simulink subsystem "Final_Project"  (R2024a)
settings: Solver=VariableStepAuto  StartTime=0.0  StopTime=10.0  RelTol=1e-3
undefined symbols (not defined in the file or in its folder): waypoints
libraries: CarMaker4SL x82
(part 4 of 4)

== matlab function Final_Project/Lib_Driving/Subsystem/MATLAB Function2 ==
  data: lat_err input; steer output; head_err input; curve_abs input; ego_v input; target_speed input; front_dist input; front_v input; mode input; lchg_done input; accel output; front_dist_lock output; park_cmd input; ego input
function [steer, accel, front_dist_lock] = controller(...
    lat_err, head_err, curve_abs, ego_v, target_speed, ...
    front_dist, front_v, mode, lchg_done, park_cmd, ego)
%#codegen

    % ============================================================
    % 기본 상수
    % ============================================================
    TS           = 0.01;
    STEER_LIM    = 0.58;
    MAX_SPEED    = 50.0;
    MODE_LCHG    = int32(1);
    MODE_PARK    = int32(2);
    KAPPA_EPS    = 1e-4;
    SPD_DEADBAND = 0.3;

    % ============================================================
    % Ego position
    % ============================================================
    ego_x = ego.Car_Fr1_tx;
    ego_y = ego.Car_Fr1_ty;

    % ============================================================
    % Parking waypoints
    % ============================================================
    L4_X     = -46.856;  L4_Y     = 15.842;
    L5_END_X =  2.617;   L5_END_Y = -35.0;

    dist_l4     = sqrt((ego_x - L4_X)^2     + (ego_y - L4_Y)^2);
    dist_to_end = sqrt((ego_x - L5_END_X)^2 + (ego_y - L5_END_Y)^2);

    % ============================================================
    % 파라미터 정의: 일반 주행 / 주차 진입
    %
    % 일반 주행부는 오류 고친 코드의 공격적인 주행 파라미터를 반영
    % 주차 진입부는 기존 주차장 버전의 저속 안정 파라미터 유지
    % ============================================================
    K_STANLEY_NRM  = 0.88;   K_STANLEY_PRK  = 0.20;
    KP_HEAD_NRM    = 0.90;   KP_HEAD_PRK    = 0.50;
    LOOK_FRONT_NRM = calcLookFront(ego_v);  LOOK_FRONT_PRK = 10.0;
    ALAT_NRM       = 3.50;   ALAT_PRK       = 1.50; %허용 횡가속도
    ATOT_NRM       = 4.00;   ATOT_PRK       = 2.00;
    MCSPD_NRM      = 7.00;   MCSPD_PRK      = 1.00;
    VREF_A_NRM     = 50.0;   VREF_A_PRK     = 2.00;
    VREF_D_NRM     = 100.0;  VREF_D_PRK     = 5.00;
    JERK_U_NRM     = 50.0;   JERK_U_PRK     = 3.00;
    JERK_D_NRM     = 60.0;   JERK_D_PRK     = 5.00;
    AMAX_NRM       = 10.0;   AMAX_PRK       = 3.00;
    DMAX_NRM       = 10.0;   DMAX_PRK       = 5.00;

    % ============================================================
    % park_cmd에 따른 파라미터 보간
    % L4에 가까워질수록 일반 주행 -> 주차 진입 파라미터로 부드럽게 전환
    % ============================================================
    FADE_FAR  = 50.0;
    FADE_NEAR = 20.0;

    if park_cmd == int32(1)
        if dist_l4 >= FADE_FAR
            r = 0.0;
        elseif dist_l4 <= FADE_NEAR
            r = 1.0;
        else
            r = (FADE_FAR - dist_l4) / (FADE_FAR - FADE_NEAR);
        end
    else
        r = 0.0;
    end

    K_STANLEY       = K_STANLEY_NRM  + r * (K_STANLEY_PRK  - K_STANLEY_NRM);
    KP_HEAD         = KP_HEAD_NRM    + r * (KP_HEAD_PRK    - KP_HEAD_NRM);
    LOOK_FRONT      = LOOK_FRONT_NRM + r * (LOOK_FRONT_PRK - LOOK_FRONT_NRM);
    A_LAT_LIMIT     = ALAT_NRM       + r * (ALAT_PRK       - ALAT_NRM);
    A_TOTAL_LIMIT   = ATOT_NRM       + r * (ATOT_PRK       - ATOT_NRM);
    MIN_CURVE_SPEED = MCSPD_NRM      + r * (MCSPD_PRK      - MCSPD_NRM);
    V_REF_ACCEL     = VREF_A_NRM     + r * (VREF_A_PRK     - VREF_A_NRM);
    V_REF_DECEL     = VREF_D_NRM     + r * (VREF_D_PRK     - VREF_D_NRM);
    JERK_UP         = JERK_U_NRM     + r * (JERK_U_PRK     - JERK_U_NRM);
    JERK_DOWN       = JERK_D_NRM     + r * (JERK_D_PRK     - JERK_D_NRM);
    ACCEL_MAX_BASE  = AMAX_NRM       + r * (AMAX_PRK       - AMAX_NRM);
    DECEL_MAX_BASE  = DMAX_NRM       + r * (DMAX_PRK       - DMAX_NRM);

    % ============================================================
    % 목표속도 결정
    % ============================================================
    if park_cmd == int32(1)

        DECEL_DIST = 25.0;
        STOP_DIST  =  2.0;

        if mode == MODE_PARK

            if dist_to_end < STOP_DIST
                ts = 0.0;
            elseif dist_to_end < DECEL_DIST
                ts = 1.4 * (dist_to_end / DECEL_DIST);
            else
                ts = 1.4;
            end

        elseif dist_l4 > FADE_NEAR

            spd_far  = 8.3;
            spd_near = 2.8;

            if dist_l4 >= FADE_FAR
                ts = spd_far;
            else
                ts = spd_far + (spd_near - spd_far) * r;
            end

        else

            ts = 2.8;

        end

    else

        ts = target_speed;

        % target_speed가 20보다 크면 km/h라고 보고 m/s로 변환
        if ts > 20.0
            ts = ts / 3.6;
        end

    end

    if ts > MAX_SPEED
        ts = MAX_SPEED;
    end

    if ts < 0.0
        ts = 0.0;
    end

    % ============================================================
    % persistent
    % ============================================================
    persistent desired_v_p accel_p did_init

    if isempty(did_init)
        desired_v_p = ego_v;
        accel_p     = 0.0;
        did_init    = true;
    end

    % ============================================================
    % 1. Stanley 조향
    % ============================================================
    v_safe = ego_v;

    if v_safe < 1.0
        v_safe = 1.0;
    end

    steer = KP_HEAD * head_err - atan2(K_STANLEY * lat_err, v_safe);

    if steer > STEER_LIM
        steer = STEER_LIM;
    elseif steer < -STEER_LIM
        steer = -STEER_LIM;
    end

    % ============================================================
    % 1-1. 끝점 추가 좌회전 블렌드
    % park_cmd=1, MODE_PARK, 끝점 5m 이내에서만 적용
    % ============================================================
    EXTRA_DIST = 5.0;
    EXTRA_RAD  = pi / 3.0;   % 60 deg

    if park_cmd == int32(1) && mode == MODE_PARK
        if dist_to_end < EXTRA_DIST && dist_to_end > 0.0
            blend = 1.0 - (dist_to_end / EXTRA_DIST);
            steer = steer + blend * EXTRA_RAD;

            % 끝점 구간만 추가 조향 허용
            if steer > EXTRA_RAD
                steer = EXTRA_RAD;
            elseif steer < -EXTRA_RAD
                steer = -EXTRA_RAD;
            end
        end
    end

    % ============================================================
    % 2. 곡률 기반 목표속도 제한
    % ============================================================
    desired_v_raw = ts;

    if curve_abs > KAPPA_EPS

        v_curve = sqrt(A_LAT_LIMIT / curve_abs);

        if v_curve < MIN_CURVE_SPEED
            v_curve = MIN_CURVE_SPEED;
        end

        if v_curve < desired_v_raw
            desired_v_raw = v_curve;
        end
    end

    % ============================================================
    % 3. ACC 앞차 감속
    % 주차 진입 중에는 비활성화
    % ============================================================
    % if park_cmd ~= int32(1)
    if mode ~= MODE_PARK

        if front_dist < LOOK_FRONT

            time_gap = 2.0;
            ACC_GAIN = 0.5;

            safe_v = front_v + (front_dist - time_gap * ego_v) * ACC_GAIN;

            if safe_v < desired_v_raw
                desired_v_raw = safe_v;
            end
        end
    end

    if desired_v_raw < 0.0
        desired_v_raw = 0.0;
    end

    % ============================================================
    % 4. 목표속도 변화율 제한
    % ============================================================
    dv = desired_v_raw - desired_v_p;

    max_dv_up = V_REF_ACCEL * TS;
    max_dv_dn = V_REF_DECEL * TS;

    if dv > max_dv_up
        desired_v_p = desired_v_p + max_dv_up;
    elseif dv < -max_dv_dn
        desired_v_p = desired_v_p - max_dv_dn;
    else
        desired_v_p = desired_v_raw;
    end

    desired_v = desired_v_p;

    % ============================================================
    % 5. 가감속
    % 주차 구간: 비례제어
    % 일반 구간: 기록 단축용 Bang-Bang
    % ============================================================
    spd_err = desired_v - ego_v;

    if park_cmd == int32(1)

        KP_SPD = 2.0;
        accel_cmd = KP_SPD * spd_err;

        if accel_cmd > ACCEL_MAX_BASE
            accel_cmd = ACCEL_MAX_BASE;
        elseif accel_cmd < -DECEL_MAX_BASE
            accel_cmd = -DECEL_MAX_BASE;
        end

    else

        if spd_err > SPD_DEADBAND
            accel_cmd = ACCEL_MAX_BASE;
        elseif spd_err < -SPD_DEADBAND
            accel_cmd = -DECEL_MAX_BASE;
        else
            accel_cmd = 0.5 * spd_err;
        end

    end

    % ============================================================
    % 6. Friction circle 기반 가속 한계
    % ============================================================
    a_lat_now = ego_v * ego_v * curve_abs;

    if a_lat_now >= A_TOTAL_LIMIT
        a_lon_avail = 0.5;
    else
        a_lon_avail = sqrt(A_TOTAL_LIMIT * A_TOTAL_LIMIT - a_lat_now * a_lat_now);

        if a_lon_avail < 0.5
            a_lon_avail = 0.5;
        end
    end

    accel_max = ACCEL_MAX_BASE;

    if a_lon_avail < accel_max
        accel_max = a_lon_avail;
    end

    if accel_cmd > accel_max
        accel_cmd = accel_max;
    end

    if accel_cmd < -DECEL_MAX_BASE
        accel_cmd = -DECEL_MAX_BASE;
    end

    % ============================================================
    % 7. Jerk 제한
    % ============================================================
    da = accel_cmd - accel_p;

    max_da_up = JERK_UP   * TS;
    max_da_dn = JERK_DOWN * TS;

    if da > max_da_up
        accel_p = accel_p + max_da_up;
    elseif da < -max_da_dn
        accel_p = accel_p - max_da_dn;
    else
        accel_p = accel_cmd;
    end

    accel = accel_p;

    % ============================================================
    % 8. front_dist_lock
    % ============================================================
    if mode == MODE_LCHG || lchg_done
        front_dist_lock = 0;
    else
        front_dist_lock = front_dist;
    end

end


function LOOK_FRONT = calcLookFront(v)
%#codegen
    v = abs(v);

    if v > 60.0
        v = v / 3.6;
    end

    % 80 km/h 기준으로 고속 구간 탐색거리 급격히 확대
    V_HIGH = 80.0 / 3.6;

    if v < V_HIGH
        LOOK_FRONT = 25.0 + 1.0 * v;
    else
        LOOK_FRONT = 25.0 + 1.0 * V_HIGH + 10.0 * (v - V_HIGH);
    end

    if LOOK_FRONT > 120.0
        LOOK_FRONT = 120.0;
    end
end

% function [steer, accel, front_dist_lock] = controller(...
%     lat_err, head_err, curve_abs, ego_v, target_speed, ...
%     front_dist, front_v, mode, lchg_done, park_cmd, ego)
% %#codegen
% 
%     TS           = 0.01;
%     STEER_LIM    = 0.58;
%     MAX_SPEED    = 50.0;
%     MODE_LCHG    = int32(1);
%     MODE_PARK    = int32(2);
%     KAPPA_EPS    = 1e-4;
%     SPD_DEADBAND = 0.3;
% 
%     ego_x = ego.Car_Fr1_tx;
%     ego_y = ego.Car_Fr1_ty;
% 
%     % Waypoint 좌표
%     L4_X     = -46.856;  L4_Y     = 15.842;
%     L5_END_X =  2.617;  L5_END_Y = -35;
% 
%     dist_l4     = sqrt((ego_x - L4_X)^2     + (ego_y - L4_Y)^2);
%     dist_to_end = sqrt((ego_x - L5_END_X)^2 + (ego_y - L5_END_Y)^2);
% 
%     % ============================================================
%     % 파라미터 정의 (일반 / 주차 최소)
%     % ============================================================
%     K_STANLEY_NRM  = 0.58;   K_STANLEY_PRK  = 0.20;
%     KP_HEAD_NRM    = 0.90;   KP_HEAD_PRK    = 0.50;
%     LOOK_FRONT_NRM = 30.0;   LOOK_FRONT_PRK = 10.0;
%     ALAT_NRM       = 3.70;   ALAT_PRK       = 1.50;
%     ATOT_NRM       = 4.00;   ATOT_PRK       = 2.00;
%     MCSPD_NRM      = 7.00;   MCSPD_PRK      = 1.00;
%     VREF_A_NRM     = 5.00;   VREF_A_PRK     = 2.00;
%     VREF_D_NRM     = 10.0;   VREF_D_PRK     = 5.00;
%     JERK_U_NRM     = 10.0;   JERK_U_PRK     = 3.00;
%     JERK_D_NRM     = 10.0;   JERK_D_PRK     = 5.00;
%     AMAX_NRM       = 10.0;   AMAX_PRK       = 3.00;
%     DMAX_NRM       = 10.0;   DMAX_PRK       = 5.00;
% 
%     % ============================================================
%     % park_cmd에 따른 파라미터 보간
%     % ============================================================
%     FADE_FAR  = 50.0;
%     FADE_NEAR = 20.0;
% 
%     if park_cmd == int32(1)
%         if dist_l4 >= FADE_FAR
%             r = 0.0;
%         elseif dist_l4 <= FADE_NEAR
%             r = 1.0;
%         else
%             r = (FADE_FAR - dist_l4) / (FADE_FAR - FADE_NEAR);
%         end
%     else
%         r = 0.0;
%     end
% 
%     K_STANLEY       = K_STANLEY_NRM  + r * (K_STANLEY_PRK  - K_STANLEY_NRM);
%     KP_HEAD         = KP_HEAD_NRM    + r * (KP_HEAD_PRK    - KP_HEAD_NRM);
%     LOOK_FRONT      = LOOK_FRONT_NRM + r * (LOOK_FRONT_PRK - LOOK_FRONT_NRM);
%     A_LAT_LIMIT     = ALAT_NRM       + r * (ALAT_PRK       - ALAT_NRM);
%     A_TOTAL_LIMIT   = ATOT_NRM       + r * (ATOT_PRK       - ATOT_NRM);
%     MIN_CURVE_SPEED = MCSPD_NRM      + r * (MCSPD_PRK      - MCSPD_NRM);
%     V_REF_ACCEL     = VREF_A_NRM     + r * (VREF_A_PRK     - VREF_A_NRM);
%     V_REF_DECEL     = VREF_D_NRM     + r * (VREF_D_PRK     - VREF_D_NRM);
%     JERK_UP         = JERK_U_NRM     + r * (JERK_U_PRK     - JERK_U_NRM);
%     JERK_DOWN       = JERK_D_NRM     + r * (JERK_D_PRK     - JERK_D_NRM);
%     ACCEL_MAX_BASE  = AMAX_NRM       + r * (AMAX_PRK       - AMAX_NRM);
%     DECEL_MAX_BASE  = DMAX_NRM       + r * (DMAX_PRK       - DMAX_NRM);
% 
%     % ============================================================
%     % 목표속도 결정
%     % ============================================================
%     if park_cmd == int32(1)
%         DECEL_DIST = 25.0;
%         STOP_DIST  =  2.0;
% 
%         if mode == MODE_PARK
%             if dist_to_end < STOP_DIST
%                 ts = 0.0;
%             elseif dist_to_end < DECEL_DIST
%                 ts = 1.4 * (dist_to_end / DECEL_DIST);
%             else
%                 ts = 1.4;
%             end
%         elseif dist_l4 > FADE_NEAR
%             spd_far  = 8.3;
%             spd_near = 2.8;
%             if dist_l4 >= FADE_FAR
%                 ts = spd_far;
%             else
%                 ts = spd_far + (spd_near - spd_far) * r;
%             end
%         else
%             ts = 2.8;
%         end
%     else
%         ts = target_speed;
%         if ts > 20.0, ts = ts / 3.6; end
%     end
% 
%     if ts > MAX_SPEED, ts = MAX_SPEED; end
%     if ts < 0.0,       ts = 0.0;       end
% 
%     % ============================================================
%     % persistent
%     % ============================================================
%     persistent desired_v_p accel_p did_init
% 
%     if isempty(did_init)
%         desired_v_p = ego_v;
%         accel_p     = 0.0;
%         did_init    = true;
%     end
% 
%     % ============================================================
%     % 1. Stanley 조향
%     % ============================================================
%     v_safe = ego_v;
%     if v_safe < 1.0, v_safe = 1.0; end
% 
%     steer = KP_HEAD * head_err - atan2(K_STANLEY * lat_err, v_safe);
% 
%     if steer >  STEER_LIM,  steer =  STEER_LIM;  end
%     if steer < -STEER_LIM,  steer = -STEER_LIM;  end
% 
%     % ============================================================
%     % 1-1. 끝점 45도 좌회전 블렌드 (park_cmd=1, MODE_PARK, 5m 이내)
%     % ============================================================
%     EXTRA_DIST = 5.0;
%     EXTRA_RAD  = pi / 3.0;   % 60 deg
% 
%     if park_cmd == int32(1) && mode == MODE_PARK
%         if dist_to_end < EXTRA_DIST && dist_to_end > 0.0
%             blend = 1.0 - (dist_to_end / EXTRA_DIST);
%             steer = steer + blend * EXTRA_RAD;
%             % 끝점 구간만 pi/4까지 허용
%             if steer >  EXTRA_RAD, steer =  EXTRA_RAD; end
%             if steer < -EXTRA_RAD, steer = -EXTRA_RAD; end
%         end
%     end
% 
%     % ============================================================
%     % 2. 곡률 기반 목표속도 제한
%     % ============================================================
%     desired_v_raw = ts;
% 
%     if curve_abs > KAPPA_EPS
%         v_curve = sqrt(A_LAT_LIMIT / curve_abs);
%         if v_curve < MIN_CURVE_SPEED, v_curve = MIN_CURVE_SPEED; end
%         if v_curve < desired_v_raw,   desired_v_raw = v_curve;   end
%     end
% 
%     % ============================================================
%     % 3. ACC 앞차 감속 (주차 중 비활성)
%     % ============================================================
%     if park_cmd ~= int32(1)
%         if front_dist < LOOK_FRONT
%             time_gap = 3.0;
%             safe_v = front_v + (front_dist - time_gap * ego_v) * 0.5;
%             if safe_v < desired_v_raw, desired_v_raw = safe_v; end
%         end
%     end
% 
%     if desired_v_raw < 0.0, desired_v_raw = 0.0; end
% 
%     % ============================================================
%     % 4. 목표속도 변화율 제한
%     % ============================================================
%     dv        = desired_v_raw - desired_v_p;
%     max_dv_up = V_REF_ACCEL * TS;
%     max_dv_dn = V_REF_DECEL * TS;
% 
%     if dv > max_dv_up
%         desired_v_p = desired_v_p + max_dv_up;
%     elseif dv < -max_dv_dn
%         desired_v_p = desired_v_p - max_dv_dn;
%     else
%         desired_v_p = desired_v_raw;
%     end
% 
%     desired_v = desired_v_p;
% 
%     % ============================================================
%     % 5. 가감속 (주차: 비례제어 / 일반: Bang-Bang)
%     % ============================================================
%     spd_err = desired_v - ego_v;
% 
%     if park_cmd == int32(1)
%         % 저속 주차 구간: 비례 제어 (bang-bang 진동 방지)
%         KP_SPD    = 2.0;
%         accel_cmd = KP_SPD * spd_err;
%         if accel_cmd >  ACCEL_MAX_BASE, accel_cmd =  ACCEL_MAX_BASE; end
%         if accel_cmd < -DECEL_MAX_BASE, accel_cmd = -DECEL_MAX_BASE; end
%     else
%         if spd_err > SPD_DEADBAND
%             accel_cmd = ACCEL_MAX_BASE;
%         elseif spd_err < -SPD_DEADBAND
%             accel_cmd = -DECEL_MAX_BASE;
%         else
%             accel_cmd = 0.5 * spd_err;
%         end
%     end
% 
%     % ============================================================
%     % 6. Friction circle
%     % ============================================================
%     a_lat_now = ego_v * ego_v * curve_abs;
% 
%     if a_lat_now >= A_TOTAL_LIMIT
%         a_lon_avail = 0.5;
%     else
%         a_lon_avail = sqrt(A_TOTAL_LIMIT^2 - a_lat_now^2);
%         if a_lon_avail < 0.5, a_lon_avail = 0.5; end
%     end
% 
%     accel_max = ACCEL_MAX_BASE;
%     if a_lon_avail < accel_max, accel_max = a_lon_avail; end
% 
%     if accel_cmd >  accel_max,       accel_cmd =  accel_max;      end
%     if accel_cmd < -DECEL_MAX_BASE,  accel_cmd = -DECEL_MAX_BASE; end
% 
%     % ============================================================
%     % 7. Jerk 제한
%     % ============================================================
%     da        = accel_cmd - accel_p;
%     max_da_up = JERK_UP   * TS;
%     max_da_dn = JERK_DOWN * TS;
% 
%     if da > max_da_up
%         accel_p = accel_p + max_da_up;
%     elseif da < -max_da_dn
%         accel_p = accel_p - max_da_dn;
%     else
%         accel_p = accel_cmd;
%     end
% 
%     accel = accel_p;
% 
%     % ============================================================
%     % 8. front_dist_lock
%     % ============================================================
%     if mode == MODE_LCHG || lchg_done
%         front_dist_lock = 0;
%     else
%         front_dist_lock = front_dist;
%     end
% 
% end

== matlab function Final_Project/Lib_Driving/Subsystem/MATLAB Function3 ==
  data: lat_err input; target_lane output int32; front_dist input; left_clear input; right_clear input; mode output; lchg_done output; park_cmd input; ego input
function [target_lane, mode, lchg_done] = decision(lat_err, front_dist, left_clear, right_clear, park_cmd, ego)
%#codegen

    % ============================================================
    % Parameters
    % ============================================================
    LCHG_TRIG_D     = 25.0;
    LAT_ARRIVED     = 0.5;

    MIN_LANE        = int32(1);
    MAX_NORMAL_LANE = int32(3);   % 일반 주행은 1~3차선만 사용
    MAX_LANE        = int32(5);   % 주차 진입 포함 전체 차선

    MODE_ACC  = int32(0);
    MODE_LCHG = int32(1);
    MODE_PARK = int32(2);

    % 샘플타임 0.01초 기준 120 step = 1.2초
    MIN_LCHG_STEP = int32(120);

    % ============================================================
    % Ego position
    % ============================================================
    ego_x = ego.Car_Fr1_tx;
    ego_y = ego.Car_Fr1_ty;

    % ============================================================
    % Parking entry waypoints
    % ============================================================
    L4_X = -46.856;  L4_Y = 15.842;
    L5_X =  -6.845;  L5_Y = 12.658;

    DIST_PREP_L3  = 50.0;
    DIST_ENTER_L4 = 20.0;
    DIST_ENTER_L5 =  8.0;

    % ============================================================
    % Persistent states
    % ============================================================
    persistent target_lane_p mode_p lchg_timer_p park_state did_init

    if isempty(did_init)
        target_lane_p = int32(2);      % 시작 차선
        mode_p        = MODE_ACC;
        lchg_timer_p  = int32(0);
        park_state    = int32(0);      % 0: 일반 주행
        did_init      = true;
    end

    % ============================================================
    % 기본 출력
    % lchg_done은 차선변경 완료 순간에만 true pulse
    % ============================================================
    target_lane = target_lane_p;
    mode        = mode_p;
    lchg_done   = false;

    % ============================================================
    % Safety clamp
    % ============================================================
    if target_lane_p < MIN_LANE
        target_lane_p = MIN_LANE;
    elseif target_lane_p > MAX_LANE
        target_lane_p = MAX_LANE;
    end

    % ============================================================
    % Distance to parking waypoints
    % ============================================================
    dist_l4 = sqrt((ego_x - L4_X)^2 + (ego_y - L4_Y)^2);
    dist_l5 = sqrt((ego_x - L5_X)^2 + (ego_y - L5_Y)^2);

    % ============================================================
    % Parking command latch
    % park_cmd는 step 신호이므로 한 번 들어오면 주차 상태머신 시작
    % ============================================================
    if park_state == int32(0)
        if park_cmd == int32(1)
            park_state = int32(1);
        end
    end

    % ============================================================
    % Parking state machine
    % ============================================================
    if park_state == int32(1)

        % L4 근처에 오기 전에 3차선으로 준비
        if mode_p ~= MODE_LCHG && dist_l4 < DIST_PREP_L3 && target_lane_p ~= int32(3)

            if target_lane_p < int32(3)
                target_lane_p = target_lane_p + int32(1);
            elseif target_lane_p > int32(3)
                target_lane_p = target_lane_p - int32(1);
            end

            mode_p       = MODE_LCHG;
            lchg_timer_p = MIN_LCHG_STEP;
        end

        % 3차선 도달 후 L4 진입 구간에서 4차선으로 이동
        if mode_p ~= MODE_LCHG && dist_l4 < DIST_ENTER_L4 && target_lane_p == int32(3)

            target_lane_p = int32(4);
            mode_p        = MODE_LCHG;
            lchg_timer_p  = MIN_LCHG_STEP;
            park_state    = int32(2);
        end

    elseif park_state == int32(2)

        % 4차선 차선변경 완료 대기
        if target_lane_p == int32(4) && mode_p ~= MODE_LCHG
            park_state = int32(3);
        end

    elseif park_state == int32(3)

        % L5 진입 지점에서 5차선으로 이동
        if mode_p ~= MODE_LCHG && dist_l5 < DIST_ENTER_L5

            target_lane_p = int32(5);
            mode_p        = MODE_LCHG;
            lchg_timer_p  = MIN_LCHG_STEP;
            park_state    = int32(4);
        end

    elseif park_state == int32(4)

        % 5차선 차선변경 완료 후 PARK 모드 진입
        if target_lane_p == int32(5) && mode_p ~= MODE_LCHG
            mode_p     = MODE_PARK;
            park_state = int32(5);
        end

    elseif park_state >= int32(5)

        mode_p = MODE_PARK;
    end

    % ============================================================
    % Parking 진행 중이면 일반 주행 로직을 타지 않음
    % ============================================================
    if park_state > int32(0)

        if mode_p == MODE_LCHG

            if lchg_timer_p > int32(0)

                lchg_timer_p = lchg_timer_p - int32(1);

            else

                if abs(lat_err) < LAT_ARRIVED
                    mode_p    = MODE_ACC;
                    lchg_done = true;
                end

            end
        end

        target_lane = target_lane_p;
        mode        = mode_p;
        return;
    end

    % ============================================================
    % 일반 주행 로직 - 오류 고친 버전 반영
    % ============================================================
    if mode_p == MODE_ACC

        if front_dist < LCHG_TRIG_D

            % 차선 번호 증가 방향 = 왼쪽
            if left_clear && target_lane_p < MAX_NORMAL_LANE

                target_lane_p = target_lane_p + int32(1);
                mode_p        = MODE_LCHG;
                lchg_timer_p  = MIN_LCHG_STEP;

            % 차선 번호 감소 방향 = 오른쪽
            elseif right_clear && target_lane_p > MIN_LANE

                target_lane_p = target_lane_p - int32(1);
                mode_p        = MODE_LCHG;
                lchg_timer_p  = MIN_LCHG_STEP;

            end
        end

    else

        % 차선변경 중 최소 시간 보장
        if lchg_timer_p > int32(0)

            lchg_timer_p = lchg_timer_p - int32(1);

        else

            % 목표 차선 중심에 충분히 가까워지면 차선변경 완료
            if abs(lat_err) < LAT_ARRIVED

                mode_p    = MODE_ACC;
                lchg_done = true;

            end
        end
    end

    % ============================================================
    % 갱신된 target_lane 바로 출력
    % 차선변경 시작 시 1 step 늦게 반영되는 것 방지
    % ============================================================
    target_lane = target_lane_p;
    mode        = mode_p;

end

% function [target_lane, mode, lchg_done] = decision(lat_err, front_dist, left_clear, right_clear, park_cmd, ego)
% %#codegen
% 
%     LCHG_TRIG_D   = 25.0;
%     LAT_ARRIVED   = 0.5;
%     MIN_LANE      = int32(1);
%     MIN_LCHG_STEP = int32(120);
% 
%     MODE_ACC  = int32(0);
%     MODE_LCHG = int32(1);
%     MODE_PARK = int32(2);
% 
%     ego_x = ego.Car_Fr1_tx;
%     ego_y = ego.Car_Fr1_ty;
% 
%     L4_X = -46.856;  L4_Y = 15.842;
%     L5_X =  -6.845;  L5_Y = 12.658;
% 
%     DIST_PREP_L3  = 50.0;
%     DIST_ENTER_L4 = 20.0;
%     DIST_ENTER_L5 =  8.0;
% 
%     persistent target_lane_p mode_p lchg_timer_p park_state did_init
% 
%     if isempty(did_init)
%         target_lane_p = int32(2);
%         mode_p        = MODE_ACC;
%         lchg_timer_p  = int32(0);
%         park_state    = int32(0);
%         did_init      = true;
%     end
% 
%     target_lane = target_lane_p;
%     mode        = mode_p;
%     lchg_done   = false;
% 
%     dist_l4 = sqrt((ego_x - L4_X)^2 + (ego_y - L4_Y)^2);
%     dist_l5 = sqrt((ego_x - L5_X)^2 + (ego_y - L5_Y)^2);
% 
%     % ============================================================
%     % 주차 상태머신
%     % ============================================================
%     if park_state == int32(0)
%         if park_cmd == int32(1)
%             park_state = int32(1);
%         end
% 
%     elseif park_state == int32(1)
%         if mode_p ~= MODE_LCHG && dist_l4 < DIST_PREP_L3 && target_lane_p ~= int32(3)
%             if target_lane_p < int32(3)
%                 target_lane_p = target_lane_p + int32(1);
%             else
%                 target_lane_p = target_lane_p - int32(1);
%             end
%             mode_p       = MODE_LCHG;
%             lchg_timer_p = MIN_LCHG_STEP;
%         end
% 
%         if mode_p ~= MODE_LCHG && dist_l4 < DIST_ENTER_L4 && target_lane_p == int32(3)
%             target_lane_p = int32(4);
%             mode_p        = MODE_LCHG;
%             lchg_timer_p  = MIN_LCHG_STEP;
%             park_state    = int32(2);
%         end
% 
%     elseif park_state == int32(2)
%         if target_lane_p == int32(4) && mode_p ~= MODE_LCHG
%             park_state = int32(3);
%         end
% 
%     elseif park_state == int32(3)
%         if mode_p ~= MODE_LCHG && dist_l5 < DIST_ENTER_L5
%             target_lane_p = int32(5);
%             mode_p        = MODE_LCHG;
%             lchg_timer_p  = MIN_LCHG_STEP;
%             park_state    = int32(4);
%         end
% 
%     elseif park_state == int32(4)
%         if target_lane_p == int32(5) && mode_p ~= MODE_LCHG
%             mode_p     = MODE_PARK;
%             park_state = int32(5);
%         end
% 
%     else
%         mode_p = MODE_PARK;
%     end
% 
%     % ============================================================
%     % 주차 진행 중: lchg_timer 관리 후 리턴
%     % ============================================================
%     if park_state > int32(0)
%         if mode_p == MODE_LCHG
%             if lchg_timer_p > int32(0)
%                 lchg_timer_p = lchg_timer_p - int32(1);
%             else
%                 if abs(lat_err) < LAT_ARRIVED
%                     mode_p    = MODE_ACC;
%                     lchg_done = true;
%                 end
%             end
%         end
%         target_lane = target_lane_p;
%         mode        = mode_p;
%         return;
%     end
% 
%     % ============================================================
%     % 일반 주행 로직
%     % ============================================================
%     if mode_p == MODE_ACC
%         if front_dist < LCHG_TRIG_D
%             if left_clear && target_lane_p < int32(3)
%                 target_lane_p = target_lane_p + int32(1);
%                 mode_p        = MODE_LCHG;
%                 lchg_timer_p  = MIN_LCHG_STEP;
%             elseif right_clear && target_lane_p > MIN_LANE
%                 target_lane_p = target_lane_p - int32(1);
%                 mode_p        = MODE_LCHG;
%                 lchg_timer_p  = MIN_LCHG_STEP;
%             end
%         end
%     else
%         if lchg_timer_p > int32(0)
%             lchg_timer_p = lchg_timer_p - int32(1);
%         else
%             if abs(lat_err) < LAT_ARRIVED
%                 mode_p    = MODE_ACC;
%                 lchg_done = true;
%             end
%         end
%     end
% 
%     target_lane = target_lane_p;
%     mode        = mode_p;
% 
% end

== matlab function Final_Project/Lib_Driving/Subsystem/MATLAB Function4 ==
  data: data input; x1 output; y1 output; x2 output; y2 output; x3 output; y3 output; x4 output; y4 output; x5 output; y5 output
function [x1,y1,x2,y2,x3,y3,x4,y4,x5,y5] = parse_lane(data)
%#codegen
    % waypoints_classified_line.xlsx 기준
    % column 1: id
    % column 2: global_x
    % column 3: global_y
    % column 4: line

    N1 = 283;
    N2 = 275;
    N3 = 266;
    N4 = 34;
    N5 = 19;

    x1 = zeros(N1, 1);
    y1 = zeros(N1, 1);

    x2 = zeros(N2, 1);
    y2 = zeros(N2, 1);

    x3 = zeros(N3, 1);
    y3 = zeros(N3, 1);

    x4 = zeros(N4, 1);
    y4 = zeros(N4, 1);

    x5 = zeros(N5, 1);
    y5 = zeros(N5, 1);

    i1 = int32(0);
    i2 = int32(0);
    i3 = int32(0);
    i4 = int32(0);
    i5 = int32(0);

    N = int32(size(data, 1));

    for k = 1:N
        lk = data(k, 4);
        xk = data(k, 2);
        yk = data(k, 3);

        if lk == 1
            if i1 < int32(N1)
                i1 = i1 + int32(1);
                x1(i1) = xk;
                y1(i1) = yk;
            end

        elseif lk == 2
            if i2 < int32(N2)
                i2 = i2 + int32(1);
                x2(i2) = xk;
                y2(i2) = yk;
            end

        elseif lk == 3
            if i3 < int32(N3)
                i3 = i3 + int32(1);
                x3(i3) = xk;
                y3(i3) = yk;
            end

        elseif lk == 4
            if i4 < int32(N4)
                i4 = i4 + int32(1);
                x4(i4) = xk;
                y4(i4) = yk;
            end

        elseif lk == 5
            if i5 < int32(N5)
                i5 = i5 + int32(1);
                x5(i5) = xk;
                y5(i5) = yk;
            end
        end
    end
end

== matlab function Final_Project/Lib_Driving/Subsystem/MATLAB Function5 ==
  data: u input; y output
function y = fcn(u)
% driving_scenario_fcn 안에서:
obs = environment.Obstacle_Info;   % 140 벡터 그대로 받음
for k = 0:27
    base = k*5;
    tx = obs(base+1);   % ← 인덱스로 바로 접근. 변환 필요 없음
    ty = obs(base+2);
    ...
end

== stateflow chart Final_Project/Chart ==
  (default) -> (junction 1)
  (junction 1) -> (junction 3) [order 1] : [mod(i,10) == 0]
      | {do_Logic_10ms;}
  (junction 1) -> (junction 7) [order 2]
  (junction 3) -> (junction 5)
  (junction 5) -> (junction 7)
  (junction 7) -> (junction 10)
  (junction 10) -> (junction 12) [order 1] : [mod(i, 50) == 0]
      | {do_Logic_50ms;}
  (junction 10) -> (junction 18) [order 2]
  (junction 12) -> (junction 16)
  (junction 16) -> (junction 18)
  (junction 18) -> (junction 25)
  (junction 25) -> (junction 27) [order 1] : [mod(i,100) == 0]
      | {do_Logic_100ms;}
  (junction 25) -> (junction 21) [order 2]
  (junction 27) -> (junction 29) : {i = 0;}
  (junction 29) -> (junction 21)
  (junction 21) -> (junction 32) : {i = i +1;}
  data: i local =0
  events: do_Logic_10ms output FUNCTION_CALL_EVENT; do_Logic_50ms output FUNCTION_CALL_EVENT; do_Logic_100ms output FUNCTION_CALL_EVENT

== matlab function Final_Project/Lib_Driving/Subsystem/MATLAB Function ==
  data: ego input; ego_lane_id output; lanes input; target_lane_fb input; lat_err output; head_err output; curve_abs output; park_cmd input
function [ego_lane_id, lat_err, head_err, curve_abs] = detector(ego, lanes, target_lane_fb, park_cmd)
%#codegen

    % ============================================================
    % 1. EgoStateBus unpack
    % ============================================================
    ego_x   = ego.Car_Fr1_tx;
    ego_y   = ego.Car_Fr1_ty;
    ego_yaw = ego.Car_Fr1_rz;

    % ============================================================
    % 2. ParsedLaneBus unpack - 5차선
    % ============================================================
    x1 = lanes.x1;  y1 = lanes.y1;
    x2 = lanes.x2;  y2 = lanes.y2;
    x3 = lanes.x3;  y3 = lanes.y3;
    x4 = lanes.x4;  y4 = lanes.y4;
    x5 = lanes.x5;  y5 = lanes.y5;

    % lane5 좌측 보정
    % 주차장 진입 버전에서 쓰던 보정 유지
    L5_OFFSET = 1.0;
    x5 = x5 + L5_OFFSET;

    % ============================================================
    % 3. 현재 ego가 가장 가까운 차선 판단
    % ============================================================
    d1 = nearest_d2(x1, y1, ego_x, ego_y);
    d2 = nearest_d2(x2, y2, ego_x, ego_y);
    d3 = nearest_d2(x3, y3, ego_x, ego_y);
    d4 = nearest_d2(x4, y4, ego_x, ego_y);
    d5 = nearest_d2(x5, y5, ego_x, ego_y);

    ego_lane_id = int32(1);
    dmin = d1;

    if d2 < dmin
        dmin = d2;
        ego_lane_id = int32(2);
    end

    if d3 < dmin
        dmin = d3;
        ego_lane_id = int32(3);
    end

    if d4 < dmin
        dmin = d4;
        ego_lane_id = int32(4);
    end

    if d5 < dmin
        ego_lane_id = int32(5);
    end

    % ============================================================
    % 4. target_lane 보호
    % ============================================================
    target_lane = int32(target_lane_fb);

    if target_lane < int32(1)
        target_lane = int32(1);
    elseif target_lane > int32(5)
        target_lane = int32(5);
    end

    % ============================================================
    % 5. 주차 진입 구간에서는 preview step 축소
    % lane4/5는 waypoint 간격/곡률 변화가 일반 차선보다 민감하므로
    % park_cmd=1일 때 더 가까운 점으로 heading을 계산
    % ============================================================
    if park_cmd == int32(1) && ...
       (target_lane == int32(4) || target_lane == int32(5))
        LOOK_STEP = int32(2);
    else
        LOOK_STEP = int32(5);
    end

    % ============================================================
    % 6. target lane 기준 lateral error / heading error / curvature 계산
    % ============================================================
    if target_lane == int32(1)

        [lat_err, head_err, curve_abs] = process_lane( ...
            x1, y1, ego_x, ego_y, ego_yaw, LOOK_STEP);

    elseif target_lane == int32(2)

        [lat_err, head_err, curve_abs] = process_lane( ...
            x2, y2, ego_x, ego_y, ego_yaw, LOOK_STEP);

    elseif target_lane == int32(3)

        [lat_err, head_err, curve_abs] = process_lane( ...
            x3, y3, ego_x, ego_y, ego_yaw, LOOK_STEP);

    elseif target_lane == int32(4)

        [lat_err, head_err, curve_abs] = process_lane( ...
            x4, y4, ego_x, ego_y, ego_yaw, LOOK_STEP);

    else

        [lat_err, head_err, curve_abs] = process_lane( ...
            x5, y5, ego_x, ego_y, ego_yaw, LOOK_STEP);

    end

end


function d2 = nearest_d2(xa, ya, ex, ey)
%#codegen

    d2 = 1e12;
    N  = int32(numel(xa));

    for i = 1:N
        dxk = xa(i) - ex;
        dyk = ya(i) - ey;
        v   = dxk*dxk + dyk*dyk;

        if v < d2
            d2 = v;
        end
    end

end


function [lat_err, head_err, curve_abs] = process_lane(xa, ya, ex, ey, eyaw, LOOK_STEP)
%#codegen

    N = int32(numel(xa));

    best_i  = int32(1);
    best_d2 = 1e12;

    % ============================================================
    % 1. ego와 가장 가까운 waypoint 찾기
    % ============================================================
    for i = 1:N
        dxk = xa(i) - ex;
        dyk = ya(i) - ey;
        v   = dxk*dxk + dyk*dyk;

        if v < best_d2
            best_d2 = v;
            best_i  = i;
        end
    end

    % ============================================================
    % 2. 경로 heading 계산
    % ============================================================
    look_i = best_i + LOOK_STEP;

    if look_i > N
        look_i = N;
    end

    if look_i > best_i

        path_yaw = atan2( ...
            ya(look_i) - ya(best_i), ...
            xa(look_i) - xa(best_i));

    elseif best_i > int32(1)

        path_yaw = atan2( ...
            ya(best_i) - ya(best_i - int32(1)), ...
            xa(best_i) - xa(best_i - int32(1)));

    else

        path_yaw = eyaw;

    end

    % ============================================================
    % 3. lateral error 계산
    % path 기준 좌표계에서 ego가 좌/우로 얼마나 떨어졌는지 계산
    % ============================================================
    dxr = ex - xa(best_i);
    dyr = ey - ya(best_i);

    lat_err = -sin(path_yaw) * dxr + cos(path_yaw) * dyr;

    % ============================================================
    % 4. heading error 계산
    % ============================================================
    head_err = path_yaw - eyaw;

    while head_err > pi
        head_err = head_err - 2.0*pi;
    end

    while head_err < -pi
        head_err = head_err + 2.0*pi;
    end

    % ============================================================
    % 5. 앞쪽 preview 곡률 계산
    % 여러 구간의 곡률 중 가장 큰 값 사용
    % ============================================================
    curve_abs = 0.0;
    STEP = int32(5);

    for kk = 0:4
        base_i = best_i + int32(kk) * STEP;

        i1 = base_i;
        i2 = base_i + STEP;
        i3 = base_i + int32(2) * STEP;

        if i1 > N
            i1 = N;
        end

        if i2 > N
            i2 = N;
        end

        if i3 > N
            i3 = N;
        end

        if i1 < i2 && i2 < i3

            yaw1 = atan2( ...
                ya(i2) - ya(i1), ...
                xa(i2) - xa(i1));

            yaw2 = atan2( ...
                ya(i3) - ya(i2), ...
                xa(i3) - xa(i2));

            dyaw = yaw2 - yaw1;

            while dyaw > pi
                dyaw = dyaw - 2.0*pi;
            end

            while dyaw < -pi
                dyaw = dyaw + 2.0*pi;
            end

            ds = sqrt( ...
                (xa(i3) - xa(i1))^2 + ...
                (ya(i3) - ya(i1))^2);

            if ds > 0.1
                kappa = abs(dyaw) / ds;

                if kappa > curve_abs
                    curve_abs = kappa;
                end
            end
        end
    end

end

% function [ego_lane_id, lat_err, head_err, curve_abs] = detector(ego, lanes, target_lane_fb, park_cmd)
% %#codegen
% 
%     ego_x   = ego.Car_Fr1_tx;
%     ego_y   = ego.Car_Fr1_ty;
%     ego_yaw = ego.Car_Fr1_rz;
% 
%     x1 = lanes.x1;  y1 = lanes.y1;
%     x2 = lanes.x2;  y2 = lanes.y2;
%     x3 = lanes.x3;  y3 = lanes.y3;
%     x4 = lanes.x4;  y4 = lanes.y4;
%     x5 = lanes.x5;  y5 = lanes.y5;
% 
%     % lane5 좌측 보정 (+x = 차량 기준 좌)
%     L5_OFFSET = 1;
%     x5 = x5 + L5_OFFSET;
% 
%     % ============================================================
%     % ego 현재 차선 판단
%     % ============================================================
%     d1 = nearest_d2(x1, y1, ego_x, ego_y);
%     d2 = nearest_d2(x2, y2, ego_x, ego_y);
%     d3 = nearest_d2(x3, y3, ego_x, ego_y);
%     d4 = nearest_d2(x4, y4, ego_x, ego_y);
%     d5 = nearest_d2(x5, y5, ego_x, ego_y);
% 
%     ego_lane_id = int32(1);
%     dmin = d1;
% 
%     if d2 < dmin, dmin = d2; ego_lane_id = int32(2); end
%     if d3 < dmin, dmin = d3; ego_lane_id = int32(3); end
%     if d4 < dmin, dmin = d4; ego_lane_id = int32(4); end
%     if d5 < dmin,             ego_lane_id = int32(5); end
% 
%     % ============================================================
%     % target_lane 보호
%     % ============================================================
%     target_lane = int32(target_lane_fb);
%     if target_lane < int32(1), target_lane = int32(1); end
%     if target_lane > int32(5), target_lane = int32(5); end
% 
%     % ============================================================
%     % lane4/5 + park_cmd=1 시 LOOK_STEP 축소
%     % ============================================================
%     if park_cmd == int32(1) && ...
%        (target_lane == int32(4) || target_lane == int32(5))
%         LOOK_STEP = int32(2);
%     else
%         LOOK_STEP = int32(5);
%     end
% 
%     % ============================================================
%     % target lane 기준 오차 계산
%     % ============================================================
%     if target_lane == int32(1)
%         [lat_err, head_err, curve_abs] = process_lane( ...
%             x1, y1, ego_x, ego_y, ego_yaw, LOOK_STEP);
% 
%     elseif target_lane == int32(2)
%         [lat_err, head_err, curve_abs] = process_lane( ...
%             x2, y2, ego_x, ego_y, ego_yaw, LOOK_STEP);
% 
%     elseif target_lane == int32(3)
%         [lat_err, head_err, curve_abs] = process_lane( ...
%             x3, y3, ego_x, ego_y, ego_yaw, LOOK_STEP);
% 
%     elseif target_lane == int32(4)
%         [lat_err, head_err, curve_abs] = process_lane( ...
%             x4, y4, ego_x, ego_y, ego_yaw, LOOK_STEP);
% 
%     else
%         [lat_err, head_err, curve_abs] = process_lane( ...
%             x5, y5, ego_x, ego_y, ego_yaw, LOOK_STEP);
%     end
% 
% end
% 
% 
% function d2 = nearest_d2(xa, ya, ex, ey)
% %#codegen
%     d2 = 1e12;
%     N  = int32(numel(xa));
%     for i = 1:N
%         dxk = xa(i) - ex;
%         dyk = ya(i) - ey;
%         v   = dxk*dxk + dyk*dyk;
%         if v < d2, d2 = v; end
%     end
% end
% 
% 
% function [lat_err, head_err, curve_abs] = process_lane(xa, ya, ex, ey, eyaw, LOOK_STEP)
% %#codegen
% 
%     N = int32(numel(xa));
% 
%     best_i  = int32(1);
%     best_d2 = 1e12;
% 
%     % ============================================================
%     % 1. 가장 가까운 waypoint
%     % ============================================================
%     for i = 1:N
%         dxk = xa(i) - ex;
%         dyk = ya(i) - ey;
%         v   = dxk*dxk + dyk*dyk;
%         if v < best_d2
%             best_d2 = v;
%             best_i  = i;
%         end
%     end
% 
%     % ============================================================
%     % 2. heading 계산
%     % ============================================================
%     look_i = best_i + LOOK_STEP;
%     if look_i > N, look_i = N; end
% 
%     if look_i > best_i
%         path_yaw = atan2( ...
%             ya(look_i) - ya(best_i), ...
%             xa(look_i) - xa(best_i));
% 
%     elseif best_i > int32(1)
%         path_yaw = atan2( ...
%             ya(best_i) - ya(best_i - int32(1)), ...
%             xa(best_i) - xa(best_i - int32(1)));
%     else
%         path_yaw = eyaw;
%     end
% 
%     % ============================================================
%     % 3. lateral error
%     % ============================================================
%     dxr = ex - xa(best_i);
%     dyr = ey - ya(best_i);
% 
%     lat_err = -sin(path_yaw) * dxr + cos(path_yaw) * dyr;
% 
%     % ============================================================
%     % 4. heading error
%     % ============================================================
%     head_err = path_yaw - eyaw;
% 
%     while head_err >  pi, head_err = head_err - 2.0*pi; end
%     while head_err < -pi, head_err = head_err + 2.0*pi; end
% 
%     % ============================================================
%     % 5. 곡률 계산
%     % ============================================================
%     curve_abs = 0.0;
%     STEP = int32(5);
% 
%     for kk = 0:4
%         base_i = best_i + int32(kk) * STEP;
%         i1 = base_i;
%         i2 = base_i + STEP;
%         i3 = base_i + int32(2) * STEP;
% 
%         if i1 > N, i1 = N; end
%         if i2 > N, i2 = N; end
%         if i3 > N, i3 = N; end
% 
%         if i1 < i2 && i2 < i3
%             yaw1 = atan2(ya(i2)-ya(i1), xa(i2)-xa(i1));
%             yaw2 = atan2(ya(i3)-ya(i2), xa(i3)-xa(i2));
% 
%             dyaw = yaw2 - yaw1;
%             while dyaw >  pi, dyaw = dyaw - 2.0*pi; end
%             while dyaw < -pi, dyaw = dyaw + 2.0*pi; end
% 
%             ds = sqrt((xa(i3)-xa(i1))^2 + (ya(i3)-ya(i1))^2);
% 
%             if ds > 0.1
%                 kappa = abs(dyaw) / ds;
%                 if kappa > curve_abs, curve_abs = kappa; end
%             end
%         end
%     end
% 
% end

== matlab function Final_Project/Lib_MissionManager/mission_manager_fcn ==
  data: ego_state input; active_scenario output; mission input Bus: MissionBus; driving_status input; tollgate_status input; parking_status input; driving_submode output; tollgate_submode output; parking_submode output
function [active_scenario, driving_submode, tollgate_submode, parking_submode] = wrapper(ego_state, mission, driving_status, tollgate_status, parking_status)
%#codegen
% Wrapper: edit functions/mission_manager_fcn.m, NOT this block
[active_scenario, driving_submode, tollgate_submode, parking_submode] = mission_manager_fcn(ego_state, mission, driving_status, tollgate_status, parking_status);
end

== matlab function Final_Project/Lib_Tollgate/tollgate_scenario_fcn ==
  data: ego_state input; trajectory_bus output; mission input Bus: MissionBus; environment input; tollgate_submode input; target_speed output; tollgate_status output; selector_ctrl output
function [trajectory_bus, target_speed, tollgate_status, selector_ctrl] = wrapper(ego_state, mission, environment, tollgate_submode)
%#codegen
% Wrapper: edit functions/tollgate_scenario_fcn.m, NOT this block
[trajectory_bus, target_speed, tollgate_status, selector_ctrl] = tollgate_scenario_fcn(ego_state, mission, environment, tollgate_submode);
end

== matlab function Final_Project/Lib_Parking/parking_scenario_fcn ==
  data: ego_state input; trajectory_bus output; mission input Bus: MissionBus; environment input; parking_submode input; target_speed output; parking_status output; selector_ctrl output
function [trajectory_bus, target_speed, parking_status, selector_ctrl] = wrapper(ego_state, mission, environment, parking_submode)
%#codegen
% Wrapper: edit functions/parking_scenario_fcn.m, NOT this block
[trajectory_bus, target_speed, parking_status, selector_ctrl] = parking_scenario_fcn(ego_state, mission, environment, parking_submode);
end

== matlab function Final_Project/Lib_VehicleController_Driving/vehicle_controller_driving_fcn ==
  data: ego_state input; steer_cmd output; active_scenario input; driving_traj input; driving_speed input; tollgate_traj input; tollgate_speed input; accel_cmd output
function [steer_cmd, accel_cmd] = wrapper(ego_state, active_scenario, driving_traj, driving_speed, tollgate_traj, tollgate_speed)
%#codegen
% Wrapper: edit functions/vehicle_controller_driving_fcn.m, NOT this block
[steer_cmd, accel_cmd] = vehicle_controller_driving_fcn(ego_state, active_scenario, driving_traj, driving_speed, tollgate_traj, tollgate_speed);
end
